simulink model "scheme4"  (R2014a)
settings: Solver=ode45  StartTime=0.0  StopTime=40  MaxStep=0.001  MinStep=0.0001  RelTol=1e-3
settings Model: Creator=User  LastModifiedBy=Анастасия

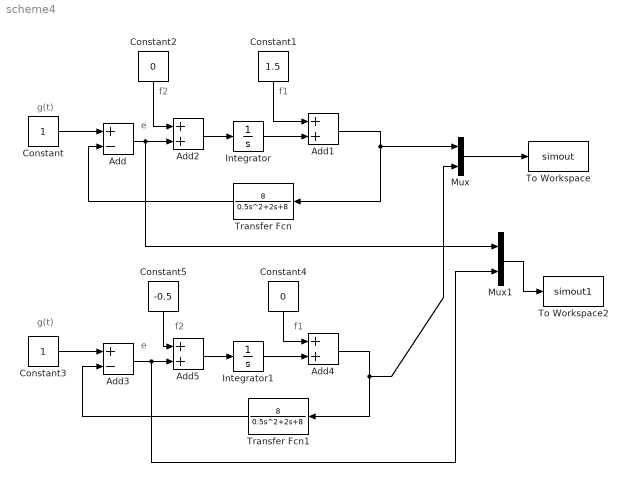
== system scheme4 ==
  note: g(t)
  note: f1
  note: f2
  note: e
  note: g(t)
  note: f1
  note: e
  note: f2
  Add : Sum  Inputs=+-
  Add{1..2,4..5} (4 alike) : Sum
  Add3 : Sum  Inputs=+-
  Constant : Constant
  Constant1 : Constant  Value=1.5
  Constant2 : Constant  Value=0
  Constant3 : Constant
  Constant4 : Constant  Value=0
  Constant5 : Constant  Value=-0.5
  Integrator : Integrator
  Integrator1 : Integrator
  Mux : Mux  Inputs=2
  Mux1 : Mux  Inputs=2
  To Workspace : ToWorkspace  VariableName=simout  SaveFormat=Timeseries  SampleTime=-1
  To Workspace2 : ToWorkspace  VariableName=simout1  SaveFormat=Timeseries  SampleTime=-1
  Transfer Fcn : TransferFcn  Numerator=8  Denominator=[0.5 2 8]
  Transfer Fcn1 : TransferFcn  Numerator=8  Denominator=[0.5 2 8]
  wires:
  Constant/1 -> Add/1
  Integrator/1 -> Add1/2
  Add2/1 -> Integrator/1
  Add/1 -> Mux1/1, Add2/2
  Constant2/1 -> Add2/1
  Constant1/1 -> Add1/1
  Constant3/1 -> Add3/1
  Add4/1 -> Mux/2, Transfer Fcn1/1
  Integrator1/1 -> Add4/2
  Add5/1 -> Integrator1/1
  Add3/1 -> Mux1/2, Add5/2
  Constant5/1 -> Add5/1
  Constant4/1 -> Add4/1
  Mux/1 -> To Workspace/1
  Mux1/1 -> To Workspace2/1
  Transfer Fcn/1 -> Add/2
  Add1/1 -> Transfer Fcn/1, Mux/1
  Transfer Fcn1/1 -> Add3/2
